simulink model "UnderstandingClasses"  (R2021a)
settings: Solver=FixedStepDiscrete  StartTime=0.0  StopTime=10.0  RelTol=1e-3
undefined symbols (not defined in the file or in its folder): D1, P
settings Model: DataDictionary=robotDD.sldd  OrderedModelArguments=off  Creator=Highlander  LastModifiedBy=Highlander

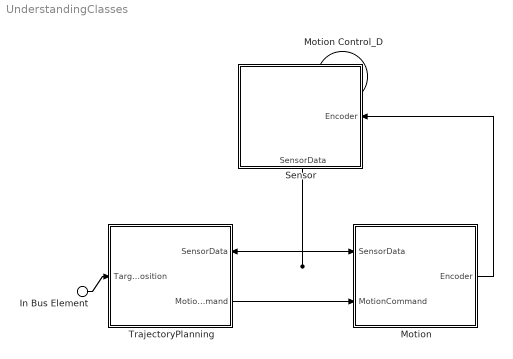
== system UnderstandingClasses ==
  In Bus Element : Inport  PortName=TargetPosition
  Motion Control_D : Inport  Port=2  OutputFunctionCall=on
  Motion : Subsystem
      settings: PortSchema="{\"entries\":[{\"content\":{\"headerSize\":26,\"margin\":15,\"minimumSpacing\":25,\"sides\":[{\"content\":{\"connectorIds\":[\"In1\",\"In2\"]},\"type\":\"ConnectorPlacement.EquallySpacedRectSide\",\"uuid\":\"7329e6a1-50ab-41f7-ba43-22322395e071\"},{\"content\":{\"connectorIds\":[\"Out1\"],\"side\":\"RIGHT\"},\"type\":\"ConnectorPlacement.EquallySpacedRectSide\",\"uuid\":\"6c016af3-0d19-4767-9069-ccb60d60668d\"},{\"content\":{\"connectorIds\":[],\"side\":\"TOP\"},\"type\":\"ConnectorPlacement.EquallySpacedRectSide\",\"uuid\":\"b1517422-2c06-4d3d-9b5e-7c012ef92d84\"}]},\"type\":\"ConnectorPlacement.EquallySpacedConnector\",\"uuid\":\"795c5afb-9669-460b-a45d-8bff0b1712ba\"}],\"packageUris\":[\"http://schema.mathworks.com/mf0/Connector/R2020b\"],\"version\":\"1.0\"}"
  Sensor : Subsystem
      settings: PortSchema="{\"entries\":[{\"content\":{\"headerSize\":26,\"margin\":15,\"minimumSpacing\":25,\"sides\":[{\"content\":{\"connectorIds\":[]},\"type\":\"ConnectorPlacement.EquallySpacedRectSide\",\"uuid\":\"7329e6a1-50ab-41f7-ba43-22322395e071\"},{\"content\":{\"connectorIds\":[\"In1\"],\"side\":\"RIGHT\"},\"type\":\"ConnectorPlacement.EquallySpacedRectSide\",\"uuid\":\"6c016af3-0d19-4767-9069-ccb60d60668d\"},{\"content\":{\"connectorIds\":[],\"side\":\"TOP\"},\"type\":\"ConnectorPlacement.EquallySpacedRectSide\",\"uuid\":\"b1517422-2c06-4d3d-9b5e-7c012ef92d84\"},{\"content\":{\"connectorIds\":[\"Out1\"],\"side\":\"BOTTOM\"},\"type\":\"ConnectorPlacement.EquallySpacedRectSide\",\"uuid\":\"c6492ffd-0cb9-4d20-a11f-28cac543c199\"}]},\"type\":\"ConnectorPlacement.EquallySpacedConnector\",\"uuid\":\"795c5afb-9669-460b-a45d-8bff0b1712ba\"}],\"packageUris\":[\"http://schema.mathworks.com/mf0/Connector/R2020b\"],\"version\":\"1.0\"}"
  TrajectoryPlanning : Subsystem
      settings: PortSchema="{\"entries\":[{\"content\":{\"headerSize\":26,\"margin\":15,\"minimumSpacing\":25,\"sides\":[{\"content\":{\"connectorIds\":[\"In1\"]},\"type\":\"ConnectorPlacement.EquallySpacedRectSide\",\"uuid\":\"7329e6a1-50ab-41f7-ba43-22322395e071\"},{\"content\":{\"connectorIds\":[\"In2\",\"Out1\"],\"side\":\"RIGHT\"},\"type\":\"ConnectorPlacement.EquallySpacedRectSide\",\"uuid\":\"6c016af3-0d19-4767-9069-ccb60d60668d\"},{\"content\":{\"connectorIds\":[],\"side\":\"TOP\"},\"type\":\"ConnectorPlacement.EquallySpacedRectSide\",\"uuid\":\"b1517422-2c06-4d3d-9b5e-7c012ef92d84\"}]},\"type\":\"ConnectorPlacement.EquallySpacedConnector\",\"uuid\":\"795c5afb-9669-460b-a45d-8bff0b1712ba\"}],\"packageUris\":[\"http://schema.mathworks.com/mf0/Connector/R2020b\"],\"version\":\"1.0\"}"
  wires:
  Sensor/1(SensorData) -> TrajectoryPlanning/2(SensorData), Motion/1(SensorData)
  TrajectoryPlanning/1(MotionCommand) -> Motion/2(MotionCommand)
  Motion/1(Encoder) -> Sensor/1(Encoder)
  In Bus Element/1 -> TrajectoryPlanning/1(TargetPosition)

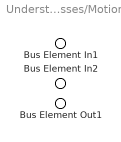
== system UnderstandingClasses/Motion ==
  Bus Element In1 : Inport  PortName=SensorData
  Bus Element In2 : Inport  Port=2  PortName=MotionCommand
  Bus Element Out1 : Outport  PortName=Encoder

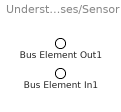
== system UnderstandingClasses/Sensor ==
  Bus Element In1 : Inport  PortName=Encoder
  Bus Element Out1 : Outport  PortName=SensorData

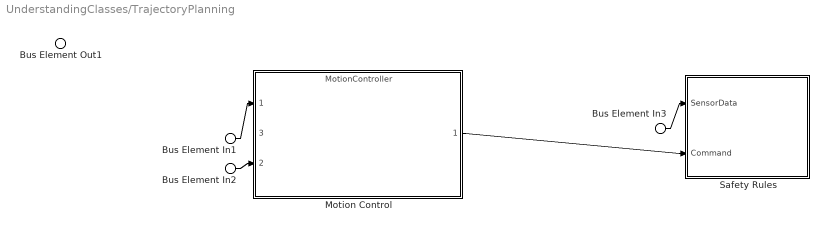
== system UnderstandingClasses/TrajectoryPlanning ==
  Bus Element In2 : Inport  PortName=TargetPosition
  Bus Element In1 : Inport  Port=2  PortName=SensorData
  Bus Element In3 : Inport  Port=2  PortName=SensorData
  Motion Control : ModelReference  ModelNameDialog=MotionController  SimulationMode=Normal  ScheduleRates=on  ModelEventPortInfo=P:D1[-2][0][0]  ModelReferenceVersion=1.4
      settings: PortSchema="{\"entries\":[{\"content\":{\"headerSize\":38,\"margin\":15,\"minimumSpacing\":25,\"sides\":[{\"content\":{\"connectorIds\":[\"In1\",\"In2\"]},\"type\":\"ConnectorPlacement.EquallySpacedRectSide\",\"uuid\":\"7329e6a1-50ab-41f7-ba43-22322395e071\"},{\"content\":{\"connectorIds\":[\"Out1\"],\"side\":\"RIGHT\"},\"type\":\"ConnectorPlacement.EquallySpacedRectSide\",\"uuid\":\"6c016af3-0d19-4767-9069-ccb60d60668d\"},{\"content\":{\"connectorIds\":[],\"side\":\"TOP\"},\"type\":\"ConnectorPlacement.EquallySpacedRectSide\",\"uuid\":\"b1517422-2c06-4d3d-9b5e-7c012ef92d84\"},{\"content\":{\"connectorIds\":[\"In3\"],\"side\":\"HIDDEN\"},\"type\":\"ConnectorPlacement.EquallySpacedRectSide\",\"uuid\":\"2423a4e0-3284-44d1-acb3-5b037d2a4f0b\"}]},\"type\":\"ConnectorPlacement.EquallySpacedConnector\",\"uuid\":\"795c5afb-9669-460b-a45d-8bff0b1712ba\"}],\"packageUris\":[\"http://schema.mathworks.com/mf0/Connector/R2020b\"],\"version\":\"1.0\"}"
  Safety Rules : Subsystem
      settings: PortSchema="{\"entries\":[{\"content\":{\"headerSize\":26,\"margin\":15,\"minimumSpacing\":25,\"sides\":[{\"content\":{\"connectorIds\":[\"In1\",\"In2\"]},\"type\":\"ConnectorPlacement.EquallySpacedRectSide\",\"uuid\":\"7329e6a1-50ab-41f7-ba43-22322395e071\"},{\"content\":{\"connectorIds\":[],\"side\":\"RIGHT\"},\"type\":\"ConnectorPlacement.EquallySpacedRectSide\",\"uuid\":\"6c016af3-0d19-4767-9069-ccb60d60668d\"},{\"content\":{\"connectorIds\":[],\"side\":\"TOP\"},\"type\":\"ConnectorPlacement.EquallySpacedRectSide\",\"uuid\":\"b1517422-2c06-4d3d-9b5e-7c012ef92d84\"}]},\"type\":\"ConnectorPlacement.EquallySpacedConnector\",\"uuid\":\"795c5afb-9669-460b-a45d-8bff0b1712ba\"}],\"packageUris\":[\"http://schema.mathworks.com/mf0/Connector/R2020b\"],\"version\":\"1.0\"}"
  Bus Element Out1 : Outport  PortName=MotionCommand
  wires:
  Bus Element In3/1 -> Safety Rules/1(SensorData)
  Bus Element In1/1 -> Motion Control/1
  Bus Element In2/1 -> Motion Control/2
  Motion Control/1 -> Safety Rules/2(Command)

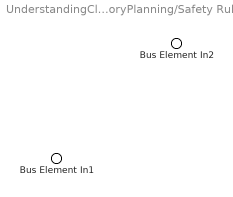
== system UnderstandingClasses/TrajectoryPlanning/Safety Rules ==
  Bus Element In2 : Inport  PortName=SensorData
  Bus Element In1 : Inport  Port=2  PortName=Command
